simulink model "Gravity_Comp"  (R2021b)
settings: Solver=VariableStepAuto  StartTime=0.0  StopTime=1  RelTol=1e-3
values from neighbouring files (symbols this model uses):
  d0 = 14    [LQRsetup.m]    (also in PIDsetup.m; datasheet.m; setup.m = 0.01228)
  mG = gc(1)    [LQRsetup.m]    (also in PIDsetup.m; datasheet.m = 1.9412)
  qG = gc(2)    [LQRsetup.m]    (also in PIDsetup.m; datasheet.m = 0.0116)
libraries: MAGLEV_components x2, spsFirstOrderFilterLib x1, slpidlib x1
settings Model: Creator=dfigu  LastModifiedBy=dfigu

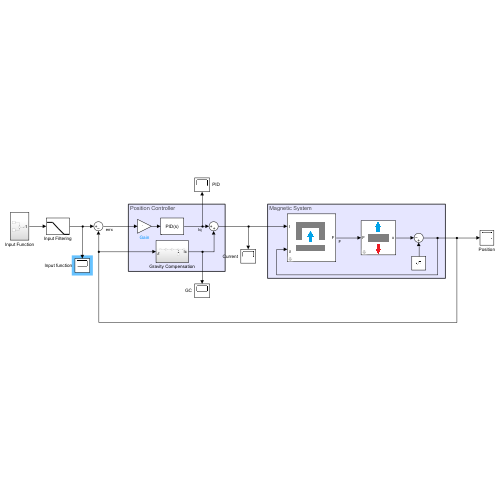
[thumbnail: Simulink's stored preview of the top-level diagram]
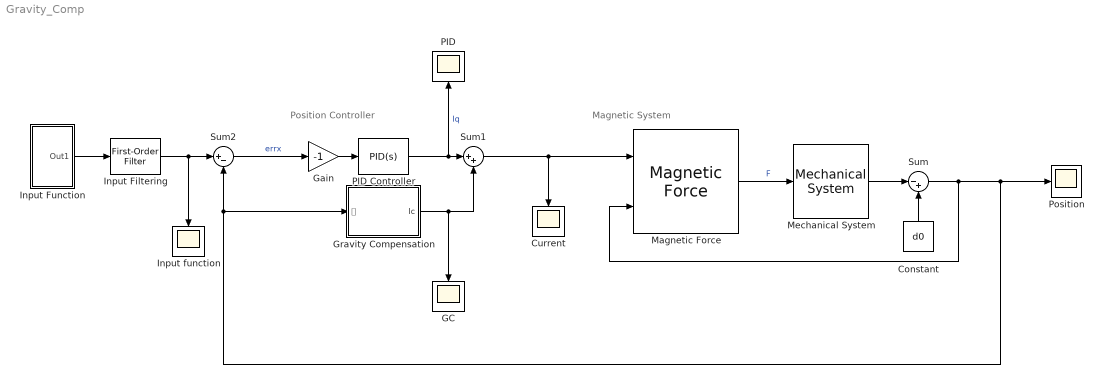
== system Gravity_Comp ==
  note: Magnetic System
  note: Position Controller
  Constant : Constant  Value=d0
  Current : Scope
  GC : Scope
  Gain : Gain  Gain=-1
  Gravity Compensation : Subsystem
  Input Filtering : spsFirstOrderFilterLib/First-Order Filter  FilterType=Lowpass  Tc=0.05  Ts=0  Initialize=on  Vac_Init=[0, 0, 60]  Vdc_Init=d0  PlotResponse=off  FreqRange="[0,  200,  1]"
  Input Function : Subsystem
  Input function : Scope
  Magnetic Force : MAGLEV_components/Magnetic Force
      link override 2-D Lookup Table: InterpMethod=Cubic spline  ExtrapMethod=Cubic spline  DiagnosticForOutOfRangeInput=Warning
  Mechanical System : MAGLEV_components/Mechanical System
  PID : Scope
  PID Controller : slpidlib/PID Controller  Controller=PID  Form=Parallel  TimeDomain=Continuous-time  UseExternalTs=off  SampleTime=-1  IntegratorMethod=Forward Euler  FilterMethod=Forward Euler  ControllerParametersSource=internal  P=0.1  I=0.3  D=0.01  UseFilter=on  N=100  TunerSelectOption=Transfer Function Based (PID Tuner App)  InitialConditionSource=internal  InitialConditionForIntegrator=0  InitialConditionForFilter=0  DifferentiatorICPrevScaledInput=0  ExternalReset=none  TrackingMode=off  Kt=1  LimitOutput=off  SatLimitsSource=internal  UpperSaturationLimit=0.4  LowerSaturationLimit=-0.4  LinearizeAsGain=on  AntiWindupMode=back-calculation  Kb=1000  POutMin=[]  POutMax=[]  IOutMin=[]  IOutMax=[]  DOutMin=[]  DOutMax=[]  NOutMin=[]  NOutMax=[]  SumOutMin=[]  SumOutMax=[]  SaturationOutMin=[]  SaturationOutMax=[]  PParamMin=[]  PParamMax=[]  IParamMin=[]  IParamMax=[]  DParamMin=[]  DParamMax=[]  NParamMin=[]  NParamMax=[]  KbParamMin=[]  KbParamMax=[]  KtParamMin=[]  KtParamMax=[]  KbOutMin=[]  KbOutMax=[]  KtOutMin=[]  KtOutMax=[]  IntegratorOutMin=[]  IntegratorOutMax=[]  FilterOutMin=[]  FilterOutMax=[]  SumI1OutMin=[]  SumI1OutMax=[]  SumI2OutMin=[]  SumI2OutMax=[]  SumI3OutMin=[]  SumI3OutMax=[]  SumI4OutMin=[]  SumI4OutMax=[]  SumDOutMin=[]  SumDOutMax=[]  DifferentiatorOutMin=[]  DifferentiatorOutMax=[]  FilterDiffOutCoefMin=[]  FilterDiffOutCoefMax=[]  ReciprocalOutMin=[]  ReciprocalOutMax=[]  SumDenOutMin=[]  SumDenOutMax=[]  SumNumOutMin=[]  SumNumOutMax=[]  DivideOutMin=[]  DivideOutMax=[]  UdiffTsProdOutMin=[]  UdiffTsProdOutMax=[]  NTsProdOutMin=[]  NTsProdOutMax=[]  UintegralTsProdOutMin=[]  UintegralTsProdOutMax=[]  UngainTsProdOutMin=[]  UngainTsProdOutMax=[]  IntegratorContinuousStateAttributes=''  IntegratorStateMustResolveToSignalObject=off  IntegratorRTWStateStorageClass=Auto  FilterContinuousStateAttributes=''  FilterStateMustResolveToSignalObject=off  FilterRTWStateStorageClass=Auto  ParallelPVariant=InternalParameters  IdealPVariant=Disabled  IVariant=InternalParameters  DVariant=InternalParameters  IntegratorVariant=Continuous  SatVariant=Disabled  AWVariant=Passthrough  PCopyVariant=Disabled  TRVariant=Disabled  FdbkBlocksVariant=Forward  IdealPFdbkVariant=Disabled  SatFdbkVariant=Disabled  DerivativeFilterVariant=ContFilter  NVariant=InternalParameters  NCopyVariant=Disabled  FilterICVariant=InternalICsFilter  IntegratorICVariant=InternalICs  ExternalResetVariant=Disabled  TRSumVariant=Passthrough  SumFdbkVariant=Disabled  SumVariant=Sum_PID  TsampFilterVariant=InternalTs  TsampNgainVariant=Passthrough  TsampIntegralVariant=Passthrough  ExternalSaturationOutDataTypeStr=Inherit: Same as second input
  Position : Scope
  Sum : Sum  Inputs=|-+
  Sum1 : Sum  Inputs=|++
  Sum2 : Sum  Inputs=|+-
  wires:
  Sum2/1 -> Gain/1  "errx"
  Input Filtering/1 -> Sum2/1, Input function/1
  Sum/1 -> Magnetic Force/2, Sum2/2, Gravity Compensation/1(𝛿), Position/1
  PID Controller/1 -> PID/1, Sum1/1  "Iq"
  Input Function/1(Out1) -> Input Filtering/1
  Gravity Compensation/1(Ic) -> Sum1/2, GC/1
  Gain/1 -> PID Controller/1
  Mechanical System/1 -> Sum/1
  Constant/1 -> Sum/2
  Magnetic Force/1 -> Mechanical System/1  "F"
  Sum1/1 -> Current/1, Magnetic Force/1

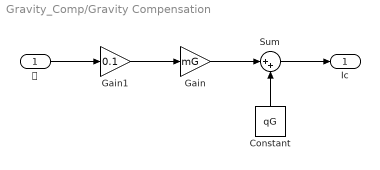
== system Gravity_Comp/Gravity Compensation ==
  𝛿 : Inport
  Constant : Constant  Value=qG
  Gain : Gain  Gain=mG
  Gain1 : Gain  Gain=0.1
  Sum : Sum  Inputs=|++
  Ic : Outport
  wires:
  Gain/1 -> Sum/1
  Sum/1 -> Ic/1
  Constant/1 -> Sum/2
  𝛿/1 -> Gain1/1
  Gain1/1 -> Gain/1

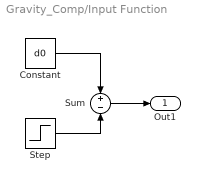
== system Gravity_Comp/Input Function ==
  Constant : Constant  Value=d0
  Step : Step  Time=0.25  After=d0/2  SampleTime=0
  Sum : Sum  Inputs=+|-
  Out1 : Outport
  wires:
  Step/1 -> Sum/2
  Sum/1 -> Out1/1
  Constant/1 -> Sum/1
